simulink model "tutorial08_masking"  (R2025a)
settings: Solver=VariableStepAuto  StartTime=0.0  StopTime=15  RelTol=1e-3
settings Model: Creator=xing2  LastModifiedBy=xing2

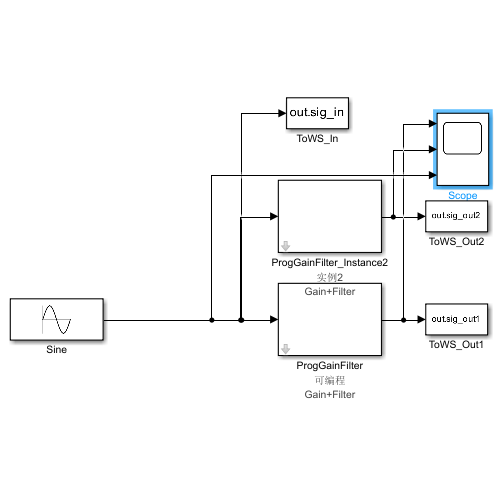
[thumbnail: Simulink's stored preview of the top-level diagram]
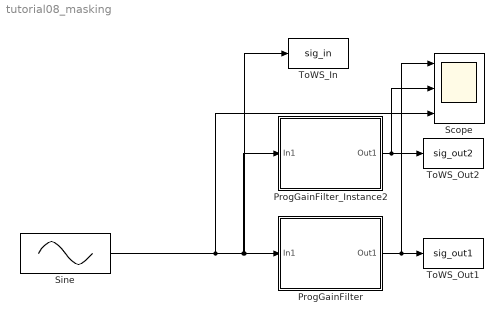
== system tutorial08_masking ==
  ProgGainFilter : Subsystem  mask{myGain=3, myTau=0.5, useFilter=on}
      mask prompts: myGain "增益 Gain 值:"; myTau "滤波时间常数 τ:"; useFilter "启用一阶滤波"
      mask help:
      | 可编程增益+一阶低通滤波器。
      | 参数：myGain - 增益倍数
      |        myTau  - 滤波时间常数 (秒)
      |        useFilter - 是否启用一阶滤波
      settings: AttributesFormatString=可编程\nGain+Filter
      mask Display: sprintf('增益=%.1f\\nτ=%.2f', myGain, myTau);
  ProgGainFilter_Instance2 : Subsystem  mask{myGain=10, myTau=2.0, useFilter=on}
      mask prompts: myGain "增益 Gain 值:"; myTau "滤波时间常数 τ:"; useFilter "启用一阶滤波"
      mask help:
      | 可编程增益+一阶低通滤波器。
      | 参数：myGain - 增益倍数
      |        myTau  - 滤波时间常数 (秒)
      |        useFilter - 是否启用一阶滤波
      settings: AttributesFormatString=实例2\nGain+Filter
      mask Display: sprintf('增益=%.1f\\nτ=%.2f', myGain, myTau);
  Scope : Scope  NumInputPorts=3
      settings: ActiveDisplayYMinimum=-26.402069506631154  ActiveDisplayYMaximum=29.375576008699685
  Sine : Sin  Amplitude=3  SampleTime=0
  ToWS_In : ToWorkspace  VariableName=sig_in  SaveFormat=Timeseries  SampleTime=-1
  ToWS_Out1 : ToWorkspace  VariableName=sig_out1  SaveFormat=Timeseries  SampleTime=-1
  ToWS_Out2 : ToWorkspace  VariableName=sig_out2  SaveFormat=Timeseries  SampleTime=-1
  wires:
  Sine/1 -> ToWS_In/1, ProgGainFilter/1(In1), ProgGainFilter_Instance2/1(In1), Scope/3
  ProgGainFilter_Instance2/1(Out1) -> Scope/2, ToWS_Out2/1
  ProgGainFilter/1(Out1) -> Scope/1, ToWS_Out1/1

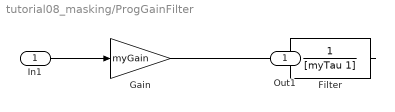
== system tutorial08_masking/ProgGainFilter ==
  In1 : Inport
  Filter : TransferFcn  Denominator=[myTau 1]
  Gain : Gain  Gain=myGain
  Out1 : Outport
  wires:
  In1/1 -> Gain/1
  Gain/1 -> Filter/1
  Filter/1 -> Out1/1

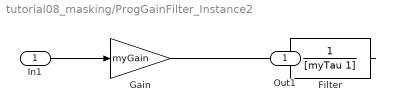
== system tutorial08_masking/ProgGainFilter_Instance2 ==
  In1 : Inport
  Filter : TransferFcn  Denominator=[myTau 1]
  Gain : Gain  Gain=myGain
  Out1 : Outport
  wires:
  Filter/1 -> Out1/1
  Gain/1 -> Filter/1
  In1/1 -> Gain/1
